simulink model "Load_Controller_V2_lowpass_13_5Hz"  (R2025a)
settings: Solver=VariableStepAuto  StartTime=0.0  StopTime=10.0  RelTol=1e-3
settings Model: Creator=Bramv  LastModifiedBy=Bramv

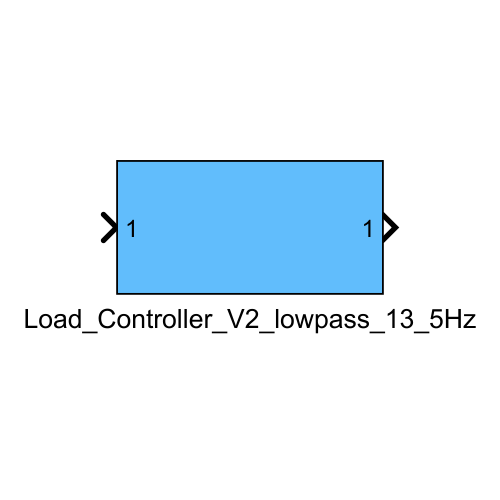
[thumbnail: Simulink's stored preview of the top-level diagram]
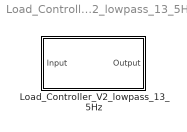
== system Load_Controller_V2_lowpass_13_5Hz ==
  Load_Controller_V2_lowpass_13_5Hz : Subsystem

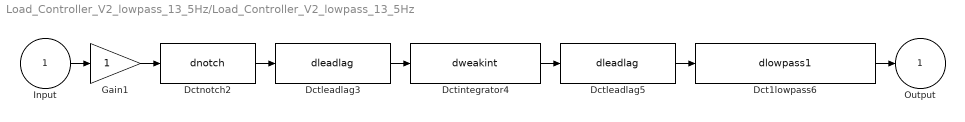
== system Load_Controller_V2_lowpass_13_5Hz/Load_Controller_V2_lowpass_13_5Hz ==
  Input : Inport
  Dct1lowpass6 : S-Function  FunctionName=dlowpass1  Parameters=f_den, 0.001  SFunctionDeploymentMode=off  EnableBusSupport=off  mask(dctools){f_den=200}
      mask prompts: f_den "Pole [Hz]"
      mask help: This block implements a discrete time 1st order lowpass filter.
      mask Display: disp('DCT 1st order lowpass')
  Dctintegrator4 : S-Function  FunctionName=dweakint  Parameters=f_num, 0.001  SFunctionDeploymentMode=off  EnableBusSupport=off  mask(dctools){f_num=0.5}
      mask prompts: f_num "Zero [Hz]"
      mask help: This block implements a discrete time weak integrator filter.
      mask Display: disp('DCT integrator')
  Dctleadlag3 : S-Function  FunctionName=dleadlag  Parameters=f_num, f_den, 0.001  SFunctionDeploymentMode=off  EnableBusSupport=off  mask(dctools){f_num=10, f_den=60}
      mask prompts: f_num "Zero [Hz]"; f_den "Pole [Hz]"
      mask help: This block implements a discrete time leadlag filter.
      mask Display: disp('DCT leadlag')
  Dctleadlag5 : S-Function  FunctionName=dleadlag  Parameters=f_num, f_den, 0.001  SFunctionDeploymentMode=off  EnableBusSupport=off  mask(dctools){f_num=18, f_den=30}
      mask prompts: f_num "Zero [Hz]"; f_den "Pole [Hz]"
      mask help: This block implements a discrete time leadlag filter.
      mask Display: disp('DCT leadlag')
  Dctnotch2 : S-Function  FunctionName=dnotch  Parameters=f_num, b_num, f_den, b_den, 0.001  SFunctionDeploymentMode=off  EnableBusSupport=off  mask(dctools){f_num=55, b_num=0.03, f_den=55, b_den=0.3}
      mask prompts: f_num "Zero [Hz]"; b_num "Damping zero [-]"; f_den "Pole [Hz]"; b_den "Damping pole [-]"
      mask help: This block implements a dicrete time 2nd order notch filter.
      mask Display: disp('DCT notch')
  Gain1 : Gain
  Output : Outport
  wires:
  Input/1 -> Gain1/1
  Gain1/1 -> Dctnotch2/1
  Dctnotch2/1 -> Dctleadlag3/1
  Dctleadlag3/1 -> Dctintegrator4/1
  Dctintegrator4/1 -> Dctleadlag5/1
  Dctleadlag5/1 -> Dct1lowpass6/1
  Dct1lowpass6/1 -> Output/1
